simulink model "sm_carousel"  (R2021b)
settings: Solver=ode15s  StartTime=0.0  StopTime=140  MaxStep=0.01  RelTol=1e-3  EnableMultiTasking=on
model workspace (MATLAB code in the model file):
  | oldDir = cd([matlabroot '/toolbox/physmod/sm/smdemos/carousel/initialization']);
  | fparams = @sm_carousel_parameters;
  | cd(oldDir);
  | fparams();
  | clear oldDir fparams;
undefined symbols (not defined in the file): Actrl, sigbuilder_block, Wctrl, X, Y, Z
libraries: sm_carousel_lib x40, sm_lib x30, nesl_utility x7
Description:
  | Fairground Carousel Ride
  | 
  | This example shows a fairground carousel ride. A torque applied to the wheel causes the carousel to rotate and a hydraulic actuator provides the force to lift the arm. The cabs are free to rotate about an axis approximately tangential to the wheel radius. When the wheel is near vertical, the centrifugal acceleration acting on the cabs (caused by the rotation of the wheel) ensures that the cabs are close to a near vertical position. Consequently, the riders are close to 'up-side-down' at the top of the rotation.
  | 
  | The acceleration at the center of the torso of a dummy is measured to show whether the ride is 'fun' and 'safe'. In addition, the hub motor power and hydraulic pressure are measured to validate the design. The control signals (reference and actual) for the hub speed and lift-arm angle are plotted to show the performance of the controllers.
settings Model: Creator=The MathWorks, Inc.  LastModifiedBy=The MathWorks, Inc.
settings SolverCC: AlgebraicLoopSolver=TrustRegion
settings DataIOCC: LimitDataPoints=on  SaveFormat=Array  SaveOutput=off  SignalLogging=off  SaveTime=off  ReturnWorkspaceOutputs=off
settings OptimizationCC: ExpressionDepthLimit=2147483647  LifeSpan=inf
settings DebuggingCC: UnderspecifiedInitializationDetection=Classic  MergeDetectMultiDrivingBlocksExec=none  SolverPrmCheckMsg=warning  StateNameClashWarn=warning  SFUnexpectedBacktrackingDiag=warning  SFNoUnconditionalDefaultTransitionDiag=warning  SFExecutionAtInitializationDiag=none  SFMachineParentedDataDiag=warning  ArithmeticOperatorsInVariantConditions=warning
settings HardwareCC: ProdBitPerPointer=32  ProdBitPerSizeT=32  ProdBitPerPtrDiffT=32  ProdLargestAtomicFloat=None  ProdIntDivRoundTo=Undefined  ProdEndianess=Unspecified  ProdWordSize=32  ProdHWDeviceType=32-bit Generic
settings ModelReferenceCC: PropagateSignalLabelsOutOfModel=off
settings SFSimCC: SimUseLocalCustomCode=off  CustomCodeUndefinedFunction=UseInterfaceOnly
settings RTWCC: RTWUseLocalCustomCode=off
settings CodeAppCC: StateflowObjectComments=on
settings GRTTargetCC: TargetLangStandard=C89/C90 (ANSI)
settings ConfigComp: CovMetricSettings=dw  CovSaveCumulativeToWorkspaceVar=on  CovSaveSingleToWorkspaceVar=on  CovExternalEMLEnable=off  CovSFcnEnable=off
settings SimscapeCC: SimscapeNormalizeSystem=off  SimscapeLogType=all  SimscapeLogSimulationStatistics=on  SimscapeLogName=simlog_sm_carousel  SimscapeLogLimitData=off
settings ConfigurationSet: Description=SimMechanics 2G
settings DiagnosticsConfigSet: SimMechanicsConflictingReferenceFrames=none
settings ExplorerConfigSet: InternalSimMechanicsExplorerSettings="<ExplorerConfiguration><canonicalview>default</canonicalview><TilePanel><TileInfo><Tiles Columns=\"1\" Count=\"1\" Rows=\"1\"><Column Left=\"2\" Weight=\"1\"/><Column Left=\"546\"/><Row Top=\"2\" Weight=\"1\"/><Row Top=\"519\"/><Tile Height=\"1\" Width=\"1\" X=\"0\" Y=\"0\"/></Tiles></TileInfo><SceneInfo><SceneViewer><BGColor><R>0.60000002384185791</R><G>0.60000002384185791</G><B>0.60000002384185791</B></BGColor><Camera><Position><X>22.971265473242269</X><Y>-23.993581807136383</Y><Z>26.226039070736011</Z></Position><Center><X>0.88896183907351589</X><Y>-1.9112781729676298</Y><Z>4.1437354365672574</Z></Center><Up><X>-0.40824829046386307</X><Y>0.40824829046386307</Y><Z>0.81649658092772615</Z></Up><Left>-9.2430366041332803</Left><Right>9.2430366041332803</Right><Bottom>-9.4834843414791639</Bottom><Top>9.4834843414791639</Top></Camera></SceneViewer></SceneInfo></TilePanel></ExplorerConfiguration>"

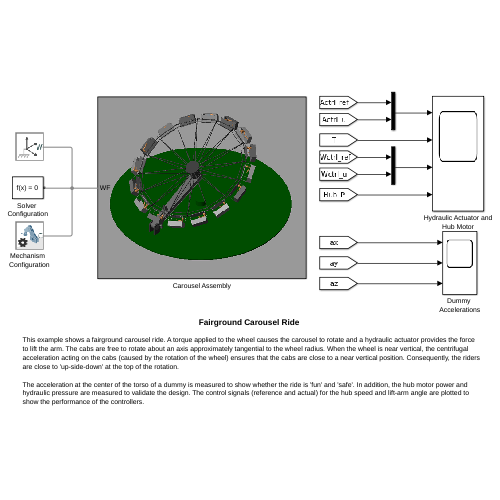
[thumbnail: Simulink's stored preview of the top-level diagram]
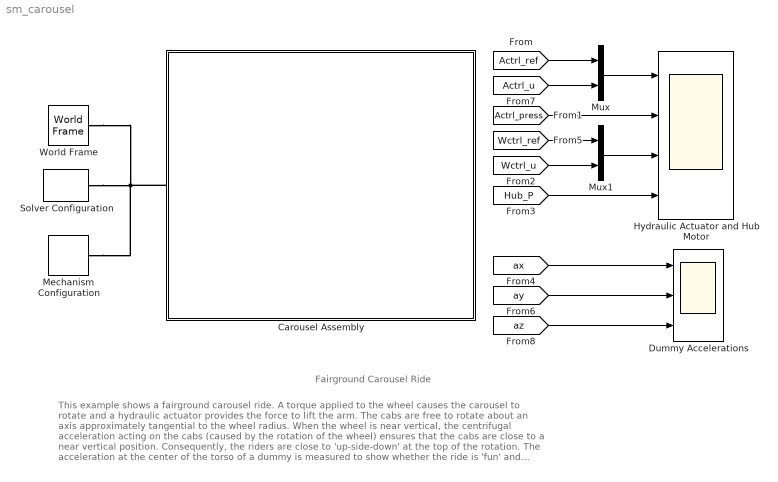
== system sm_carousel ==
  note: This example shows a fairground carousel ride. A torque applied to the wheel causes the carousel to rotate and a hydraulic actuator provides the force
      | to lift the arm. The cabs are free to rotate about an axis approximately tangential to the wheel radius. When the wheel is near vertical, the centrifugal
      | acceleration acting on the cabs (caused by the rotation of the wheel) ensures that the cabs are close to a near vertical position. Consequently, the riders
      | are close to 'up-side-down' at the top of the rotation.
      |
      | The acceleration at the center of the torso of a dummy is measured to show whether the ride is 'fun' and 'safe'. In addition, the hub motor power and
      | hydraulic pressure are measured to validate the design. The control signals (reference and actual) for the hub speed and lift-arm angle are plotted to
      | show the performance of the controllers.
  note: Fairground Carousel Ride
  Carousel Assembly : Subsystem
      mask Display:
      | image(fullfile(matlabroot,'toolbox','physmod','sm','smdemos','carousel','images','sm_carousel.png'));
      | port_label('lconn',1,'WF');
  Dummy Accelerations : Scope  NumInputPorts=3
  Hydraulic Actuator and Hub Motor : Scope  NumInputPorts=4
  Mechanism Configuration : sm_lib/Utilities/Mechanism Configuration  UniformGravity=Constant  GravityVector=[0 0 -9.81]  GravityUnits=m/s^2  LinearizationDelta=0.001  JointModeTransitionNonlinearIterations=2
  Mux : Mux  Inputs=2
  Mux1 : Mux  Inputs=2
  Solver Configuration : nesl_utility/Solver Configuration  PhysicalDomain=network_engine_domain  SubClassName=solver  LeftPortType=input  RightPortType=generic  Tones=[]  Harmonics=[]  SimulateNoise=off  Profile=off  UseLocalSampling=off  EnableSwitchedLinearOptims=on  FrequencyDomain=off  UseCCode=off  RelTol=0.001  AbsTol=1e-06  MinStep=1e-09  ToWorkspace=off  RevertToSquareIcSolve=off  NumHomotopyIterations=100  PhasorMode=off  PhasorModeNumHarmonics=1  DoDC=off  ResidualTolerance=1e-9  UseLocalSolver=off  LocalSolverChoice=NE_BACKWARD_EULER_ADVANCER  LocalSolverSampleTime=.001  DoFixedCost=off  MaxNonlinIter=3  MaxModeIter=2  ComputeImpulses=off  ImpulseIterations=2  LinearAlgebra=Sparse  EquationFormulation=NE_TIME_EF  DelaysMemoryBudget=1024  AutomaticFiltering=on  FilteringTimeConstant=0.001  PartitionStorageMethod=AS_NEEDED  PartitionMemoryBudget=1024  PartitionMethod=FAST
      settings: SourceProductBaseCode=PW,SS
  World Frame : sm_lib/Frames and Transforms/World Frame
  wires:
  [Actrl_ref] -> Mux/1
  [Actrl_u] -> Mux/2
  Mux/1 -> Hydraulic Actuator and Hub Motor/1
  [Wctrl_ref] -> Mux1/1
  [Wctrl_u] -> Mux1/2
  Mux1/1 -> Hydraulic Actuator and Hub Motor/3
  [Actrl_press] -> Hydraulic Actuator and Hub Motor/2
  [Hub_P] -> Hydraulic Actuator and Hub Motor/4
  [az] -> Dummy Accelerations/3
  [ay] -> Dummy Accelerations/2
  [ax] -> Dummy Accelerations/1
  connections:
  Solver Configuration/RConn1 -- Mechanism Configuration/RConn1 -- Carousel Assembly/LConn1 -- World Frame/RConn1

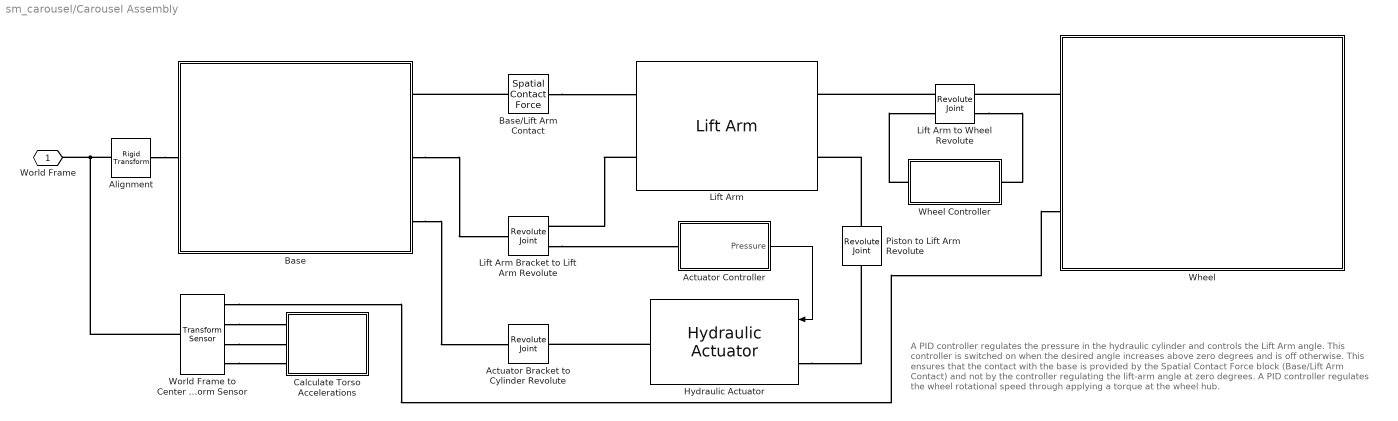
== system sm_carousel/Carousel Assembly ==
  note: A PID controller regulates the pressure in the hydraulic cylinder and controls the Lift Arm angle. This controller is switched on when the desired angle increases above zero degrees and is off otherwise. This ensures that the contact with the base is provided by the Spatial Contact Force block (Base/Lift Arm Contact) and not by the controller regulating the lift-arm angle at zero degrees. A PID controller regulates the wheel rotational speed through applying a torque at the wheel hub.
  Actuator Bracket to Cylinder Revolute : sm_lib/Joints/Revolute Joint  JointMode=Normal  SenseConstraintForce=off  SenseConstraintForceX=off  SenseConstraintForceY=off  SenseConstraintForceZ=off  SenseConstraintTorque=off  SenseConstraintTorqueX=off  SenseConstraintTorqueY=off  SenseConstraintTorqueZ=off  SenseTotalForce=off  SenseTotalForceX=off  SenseTotalForceY=off  SenseTotalForceZ=off  SenseTotalTorque=off  SenseTotalTorqueX=off  SenseTotalTorqueY=off  SenseTotalTorqueZ=off  CompositeWrenchDir=FollowerOnBase  CompositeWrenchFrame=BaseFrame  EquilibriumPosition=0  EquilibriumPositionUnits=deg  SpringStiffness=0  SpringStiffnessUnits=N*m/deg  DampingCoefficient=0  DampingCoefficientUnits=N*m/(deg/s)  TorqueActuationMode=NoTorque  MotionActuationMode=ComputedMotion  SensePosition=off  SenseVelocity=off  SenseAcceleration=off  SenseTorqueForce=off  SenseLowerLimitTorqueForce=off  SenseUpperLimitTorqueForce=off  LowerLimitSpecify=off  LowerLimitBound=-90  LowerLimitBoundUnits=deg  LowerLimitStiffness=1e4  LowerLimitStiffnessUnits=N*m/deg  LowerLimitDamping=10  LowerLimitDampingUnits=N*m/(deg/s)  LowerLimitTransitionRegionWidth=0.1  LowerLimitTransitionRegionWidthUnits=deg  UpperLimitSpecify=off  UpperLimitBound=90  UpperLimitBoundUnits=deg  UpperLimitStiffness=1e4  UpperLimitStiffnessUnits=N*m/deg  UpperLimitDamping=10  UpperLimitDampingUnits=N*m/(deg/s)  UpperLimitTransitionRegionWidth=0.1  UpperLimitTransitionRegionWidthUnits=deg  PositionTargetSpecify=off  PositionTargetPriority=High  PositionTargetValue=0  PositionTargetValueUnits=deg  VelocityTargetSpecify=off  VelocityTargetPriority=High  VelocityTargetValue=0  VelocityTargetValueUnits=deg/s
  Actuator Controller : Subsystem
      mask Display:
      | port_label('lconn',1,'q');
      | port_label('output',1,'P');
  Alignment : sm_lib/Frames and Transforms/Rigid Transform  TranslationMethod=None  TranslationStandardOffset=0  TranslationLengthUnit=m  TranslationStandardAxis=+Z  TranslationCartesianOffset=[0 0 0]  TranslationROffset=0  TranslationROffsetUnits=m  TranslationZOffset=0  TranslationZOffsetUnits=m  TranslationThetaOffset=0  TranslationThetaOffsetUnits=deg  RotationMethod=AlignedAxes  RotationAngleUnits=deg  RotationStandardAxis=+Z  RotationAngle=0  RotationArbitraryAxis=[0 0 1]  FollAlignAxisA=+X  BaseAlignAxisA=+Y  FollAlignAxisB=+Z  BaseAlignAxisB=+Z  RotationSequenceAxes=FollowerAxes  RotationSequence=XYX  RotationSequenceAngles=[0 0 0]  RotationSequenceAnglesUnits=deg  RotationMatrix=[1 0 0; 0 1 0; 0 0 1]
  Base : Subsystem
      mask Display:
      | image(fullfile(matlabroot,'toolbox','physmod','sm','smdemos','carousel','images','sm_carousel_base.png'));
      | port_label('lconn',1,'WF');
      | port_label('rconn',1,'CG');
      | port_label('rconn',2,'RA');
      | port_label('rconn',3,'CB');
  Base/Lift Arm Contact : sm_lib/Forces and Torques/Spatial Contact Force  CoefficientOfDynamicFriction=0.3  CoefficientOfStaticFriction=0.5  SenseContactBaseRotation=off  SenseContactBaseTranslation=off  NormalDamping=Base.b  NormalDampingUnits=N/(m/s)  SenseContactFollowerRotation=off  SenseContactFollowerTranslation=off  SenseContactSignal=off  NormalStiffness=Base.k  NormalStiffnessUnits=N/m  FrictionalCriticalVelocity=1e-3  FrictionalCriticalVelocityUnits=m/s  ZeroCrossDetectContactStartAndEnd=off  FrictionType=None  SenseFrictionalForceMagnitude=off  SenseNormalForceMagnitude=off  NormalForceType=SmoothSpringDamper  SenseNormalVelocity=off  SenseSeparationDistance=off  SenseTangentialVelocity=off  SenseTangentialVelocityMagnitude=off  NormalTransitionRegionWidth=1e-4  NormalTransitionRegionWidthUnits=m
  Calculate Torso Accelerations : Subsystem
      mask Display:
      | port_label('lconn',1,'ax');
      | port_label('lconn',2,'ay');
      | port_label('lconn',3,'az');
  Hydraulic Actuator : sm_carousel_lib/Hydraulic Actuator  Lcyl=Actuator.cyl.Lcyl  Rcyl=Actuator.cyl.Rcyl  Lbase=Actuator.cyl.Lbase  Wbase=Actuator.cyl.Wbase  Rbp=Actuator.cyl.Rbp  Lpist=Actuator.pist.Lpist  Rpist=Actuator.pist.Rpist  Whead=Actuator.pist.Whead  Lhead=Actuator.pist.Lhead  Rhp=Actuator.pist.Rhp  cylColor=Actuator.Mat.cylColor  rhoCyl=Actuator.Mat.rhoCyl  pistColor=Actuator.Mat.pistColor  rhoPist=Actuator.Mat.rhoPist  connColor=Actuator.Mat.connColor  rhoConn=Actuator.Mat.rhoConn
      settings: SourceProductBaseCode=MS
  Lift Arm : sm_carousel_lib/Lift Arm  LiftArmLength=liftArm.ArmMain.ArmLength  rootWidth=liftArm.ArmMain.ArmRootWidth  ArmRadius=liftArm.ArmMain.ArmRadius  LiftArmDepth=liftArm.ArmMain.ArmDepth  LiftArmLip=liftArm.ArmMain.ArmLip  plateThickness=liftArm.ArmMain.Thickness  Hbracket=liftArm.AB.H  Wbracket=liftArm.AB.W  Tbracket=liftArm.AB.T  Dbracket=liftArm.AB.D  Hhole=liftArm.AB.HO  Rhole=liftArm.AB.HR  PistonBracketOffset=liftArm.AB.BO  TopHoleOffset=liftArm.TopPlate.HoleOffset  TopHoleW=liftArm.TopPlate.HoleWidth  TopHoleL=liftArm.TopPlate.HoleLength  BottomHoleOffset=liftArm.BottomPlate.HoleOffset  BottomHoleW=liftArm.BottomPlate.HoleWidth  BottomHoleL=liftArm.BottomPlate.HoleLength  rhoLiftArm=liftArm.ArmMain.Density  LiftArmColor=liftArm.ArmMain.Color
      settings: SourceProductBaseCode=MS
  Lift Arm Bracket to Lift Arm Revolute : sm_lib/Joints/Revolute Joint  JointMode=Normal  SenseConstraintForce=off  SenseConstraintForceX=off  SenseConstraintForceY=off  SenseConstraintForceZ=off  SenseConstraintTorque=off  SenseConstraintTorqueX=off  SenseConstraintTorqueY=off  SenseConstraintTorqueZ=off  SenseTotalForce=off  SenseTotalForceX=off  SenseTotalForceY=off  SenseTotalForceZ=off  SenseTotalTorque=off  SenseTotalTorqueX=off  SenseTotalTorqueY=off  SenseTotalTorqueZ=off  CompositeWrenchDir=FollowerOnBase  CompositeWrenchFrame=BaseFrame  EquilibriumPosition=0  EquilibriumPositionUnits=deg  SpringStiffness=0  SpringStiffnessUnits=N*m/deg  DampingCoefficient=0  DampingCoefficientUnits=N*m/(deg/s)  TorqueActuationMode=NoTorque  MotionActuationMode=ComputedMotion  SensePosition=on  SenseVelocity=off  SenseAcceleration=off  SenseTorqueForce=off  SenseLowerLimitTorqueForce=off  SenseUpperLimitTorqueForce=off  LowerLimitSpecify=off  LowerLimitBound=-90  LowerLimitBoundUnits=deg  LowerLimitStiffness=1e4  LowerLimitStiffnessUnits=N*m/deg  LowerLimitDamping=10  LowerLimitDampingUnits=N*m/(deg/s)  LowerLimitTransitionRegionWidth=0.1  LowerLimitTransitionRegionWidthUnits=deg  UpperLimitSpecify=off  UpperLimitBound=90  UpperLimitBoundUnits=deg  UpperLimitStiffness=1e4  UpperLimitStiffnessUnits=N*m/deg  UpperLimitDamping=10  UpperLimitDampingUnits=N*m/(deg/s)  UpperLimitTransitionRegionWidth=0.1  UpperLimitTransitionRegionWidthUnits=deg  PositionTargetSpecify=on  PositionTargetPriority=High  PositionTargetValue=liftArm.Revolute.InitAngle  PositionTargetValueUnits=deg  VelocityTargetSpecify=off  VelocityTargetPriority=High  VelocityTargetValue=0  VelocityTargetValueUnits=deg/s
  Lift Arm to Wheel Revolute : sm_lib/Joints/Revolute Joint  JointMode=Normal  SenseConstraintForce=off  SenseConstraintForceX=off  SenseConstraintForceY=off  SenseConstraintForceZ=off  SenseConstraintTorque=off  SenseConstraintTorqueX=off  SenseConstraintTorqueY=off  SenseConstraintTorqueZ=off  SenseTotalForce=off  SenseTotalForceX=off  SenseTotalForceY=off  SenseTotalForceZ=off  SenseTotalTorque=off  SenseTotalTorqueX=off  SenseTotalTorqueY=off  SenseTotalTorqueZ=off  CompositeWrenchDir=FollowerOnBase  CompositeWrenchFrame=BaseFrame  EquilibriumPosition=0  EquilibriumPositionUnits=deg  SpringStiffness=0  SpringStiffnessUnits=N*m/deg  DampingCoefficient=0  DampingCoefficientUnits=N*m/(deg/s)  TorqueActuationMode=InputTorque  MotionActuationMode=ComputedMotion  SensePosition=off  SenseVelocity=on  SenseAcceleration=off  SenseTorqueForce=off  SenseLowerLimitTorqueForce=off  SenseUpperLimitTorqueForce=off  LowerLimitSpecify=off  LowerLimitBound=-90  LowerLimitBoundUnits=deg  LowerLimitStiffness=1e4  LowerLimitStiffnessUnits=N*m/deg  LowerLimitDamping=10  LowerLimitDampingUnits=N*m/(deg/s)  LowerLimitTransitionRegionWidth=0.1  LowerLimitTransitionRegionWidthUnits=deg  UpperLimitSpecify=off  UpperLimitBound=90  UpperLimitBoundUnits=deg  UpperLimitStiffness=1e4  UpperLimitStiffnessUnits=N*m/deg  UpperLimitDamping=10  UpperLimitDampingUnits=N*m/(deg/s)  UpperLimitTransitionRegionWidth=0.1  UpperLimitTransitionRegionWidthUnits=deg  PositionTargetSpecify=off  PositionTargetPriority=High  PositionTargetValue=0  PositionTargetValueUnits=deg  VelocityTargetSpecify=off  VelocityTargetPriority=High  VelocityTargetValue=0  VelocityTargetValueUnits=deg/s
  Piston to Lift Arm Revolute : sm_lib/Joints/Revolute Joint  JointMode=Normal  SenseConstraintForce=off  SenseConstraintForceX=off  SenseConstraintForceY=off  SenseConstraintForceZ=off  SenseConstraintTorque=off  SenseConstraintTorqueX=off  SenseConstraintTorqueY=off  SenseConstraintTorqueZ=off  SenseTotalForce=off  SenseTotalForceX=off  SenseTotalForceY=off  SenseTotalForceZ=off  SenseTotalTorque=off  SenseTotalTorqueX=off  SenseTotalTorqueY=off  SenseTotalTorqueZ=off  CompositeWrenchDir=FollowerOnBase  CompositeWrenchFrame=BaseFrame  EquilibriumPosition=0  EquilibriumPositionUnits=deg  SpringStiffness=0  SpringStiffnessUnits=N*m/deg  DampingCoefficient=0  DampingCoefficientUnits=N*m/(deg/s)  TorqueActuationMode=NoTorque  MotionActuationMode=ComputedMotion  SensePosition=off  SenseVelocity=off  SenseAcceleration=off  SenseTorqueForce=off  SenseLowerLimitTorqueForce=off  SenseUpperLimitTorqueForce=off  LowerLimitSpecify=off  LowerLimitBound=-90  LowerLimitBoundUnits=deg  LowerLimitStiffness=1e4  LowerLimitStiffnessUnits=N*m/deg  LowerLimitDamping=10  LowerLimitDampingUnits=N*m/(deg/s)  LowerLimitTransitionRegionWidth=0.1  LowerLimitTransitionRegionWidthUnits=deg  UpperLimitSpecify=off  UpperLimitBound=90  UpperLimitBoundUnits=deg  UpperLimitStiffness=1e4  UpperLimitStiffnessUnits=N*m/deg  UpperLimitDamping=10  UpperLimitDampingUnits=N*m/(deg/s)  UpperLimitTransitionRegionWidth=0.1  UpperLimitTransitionRegionWidthUnits=deg  PositionTargetSpecify=off  PositionTargetPriority=High  PositionTargetValue=0  PositionTargetValueUnits=deg  VelocityTargetSpecify=off  VelocityTargetPriority=High  VelocityTargetValue=0  VelocityTargetValueUnits=deg/s
  Wheel : Subsystem
      mask Display:
      | image(fullfile(matlabroot,'toolbox','physmod','sm','smdemos','carousel','images','sm_carousel_wheel_assembly.png'));
      | port_label('lconn',2,'CT');
      | port_label('lconn',1,'HA');
  Wheel Controller : Subsystem
      mask Display:
      | port_label('rconn',1,'T');
      | port_label('lconn',1,'w');
  World Frame to Center Torso XForm Sensor : sm_lib/Frames and Transforms/Transform Sensor  MeasurementFrame=NonRotatingFollower  SenseAngle=off  SenseAxis=off  SenseAngle1=off  SenseAngle2=off  SenseAngle3=off  SenseQ=off  SenseR=off  SenseOmegaX=off  SenseOmegaY=off  SenseOmegaZ=off  SenseOmega1=off  SenseOmega2=off  SenseOmega3=off  SenseQDot=off  SenseRDot=off  SenseAlphaX=off  SenseAlphaY=off  SenseAlphaZ=off  SenseAlpha1=off  SenseAlpha2=off  SenseAlpha3=off  SenseQDDot=off  SenseRDDot=off  SenseX=off  SenseY=off  SenseZ=off  SenseRad=off  SenseAzim=off  SenseDist=off  SenseInc=off  SenseXDot=off  SenseYDot=off  SenseZDot=off  SenseRadDot=off  SenseAzimDot=off  SenseDistDot=off  SenseIncDot=off  SenseXDDot=on  SenseYDDot=on  SenseZDDot=on  SenseRadDDot=off  SenseAzimDDot=off  SenseDistDDot=off  SenseIncDDot=off
  World Frame : PMIOPort  Side=Left
  wires:
  Actuator Controller/1(Pressure) -> Hydraulic Actuator/1
  connections:
  Base/RConn3 -- Actuator Bracket to Cylinder Revolute/LConn1
  Lift Arm Bracket to Lift Arm Revolute/RConn2 -- Actuator Controller/LConn1
  Wheel Controller/RConn1 -- Lift Arm to Wheel Revolute/LConn2
  Base/RConn2 -- Lift Arm Bracket to Lift Arm Revolute/LConn1
  Lift Arm/LConn2 -- Lift Arm Bracket to Lift Arm Revolute/RConn1
  Hydraulic Actuator/LConn1 -- Piston to Lift Arm Revolute/LConn1
  Lift Arm to Wheel Revolute/LConn1 -- Lift Arm/RConn1
  Piston to Lift Arm Revolute/RConn1 -- Lift Arm/RConn2
  Hydraulic Actuator/RConn1 -- Actuator Bracket to Cylinder Revolute/RConn1
  World Frame to Center Torso XForm Sensor/RConn1 -- Wheel/LConn2
  World Frame to Center Torso XForm Sensor/LConn1 -- Alignment/LConn1 -- World Frame/RConn1
  Lift Arm to Wheel Revolute/RConn2 -- Wheel Controller/LConn1
  World Frame to Center Torso XForm Sensor/RConn2 -- Calculate Torso Accelerations/LConn1
  World Frame to Center Torso XForm Sensor/RConn3 -- Calculate Torso Accelerations/LConn2
  World Frame to Center Torso XForm Sensor/RConn4 -- Calculate Torso Accelerations/LConn3
  Wheel/LConn1 -- Lift Arm to Wheel Revolute/RConn1
  Alignment/RConn1 -- Base/LConn1
  Base/Lift Arm Contact/LConn1 -- Base/RConn1
  Base/Lift Arm Contact/RConn1 -- Lift Arm/LConn1

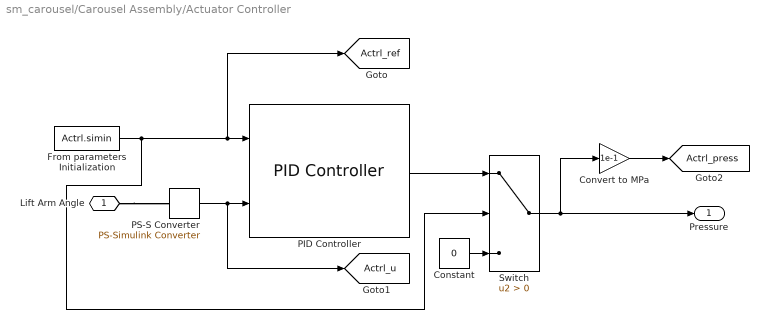
== system sm_carousel/Carousel Assembly/Actuator Controller ==
  Constant : Constant  Value=0
  Convert to MPa : Gain  Gain=1e-1
  From parameters Initialization : FromWorkspace  VariableName=Actrl.simin
  PID Controller : sm_carousel_lib/PID Controller  Kp=Actrl.kp  Ki=Actrl.ki  Kd=Actrl.kd  N=Actrl.N
      settings: SourceProductBaseCode=MS
  PS-S Converter : nesl_utility/PS-Simulink Converter  PhysicalDomain=network_engine_domain  SubClassName=ps_output  LeftPortType=input  RightPortType=output  PseudoPeriodic=off  Frequencies=[]  Unit=deg  AffineConversion=off
      settings: SourceProductBaseCode=PW,SS
  Switch : Switch  Criteria=u2 > Threshold
  Lift Arm Angle : PMIOPort  Side=Left
  Pressure : Outport
  tag scope: Actrl_press=global, Actrl_ref=global, Actrl_u=global
  wires:
  PS-S Converter/1 -> PID Controller/2, [Actrl_u]
  Convert to MPa/1 -> [Actrl_press]
  Switch/1 -> Pressure/1, Convert to MPa/1
  PID Controller/1 -> Switch/1
  Constant/1 -> Switch/3
  From parameters Initialization/1 -> Switch/2, [Actrl_ref], PID Controller/1
  connections:
  Lift Arm Angle/RConn1 -- PS-S Converter/LConn1

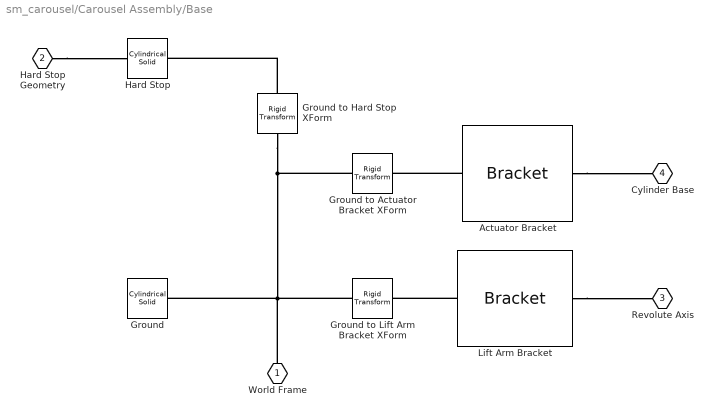
== system sm_carousel/Carousel Assembly/Base ==
  Actuator Bracket : sm_carousel_lib/Bracket  Hbracket=Base.AB.H  Wbracket=Base.AB.W  Tbracket=Base.AB.T  Dbracket=Base.AB.D  Hhole=Base.AB.HH  Rhole=Base.AB.RH  rhoBracket=Base.AB.RHO  bracketColor=Base.AB.COLOR
      settings: SourceProductBaseCode=MS
  Ground : sm_lib/Body Elements/Cylindrical Solid  GraphicAmbientColor=[0.15 0.15 0.15 1.0]  BasedOnType=Density  CenterOfMass=[0 0 0]  CenterOfMassUnits=m  GraphicDiffuseColor=Base.Color  CylinderLength=Base.Ground.t  CylinderLengthUnits=m  CylinderRadius=Base.Ground.r  CylinderRadiusUnits=m  Density=1000  DensityUnits=kg/(m^3)  DoExposeReferenceFrame=on  GraphicEmissiveColor=[0.0 0.0 0.0 1.0]  ExportEntireGeometry=off  SerializedFrames=<Frames/>  MarkerShape=Sphere  MarkerSize=10  GraphicType=FromGeometry  InertiaType=CalculateFromGeometry  Mass=1  MassUnits=kg  MomentsOfInertia=[1 1 1]  MomentsOfInertiaUnits=kg*m^2  GraphicOpacity=1.0  ProductsOfInertia=[0 0 0]  ProductsOfInertiaUnits=kg*m^2  GraphicShininess=75  GraphicSpecularColor=[0.5 0.5 0.5 1.0]  GraphicVisPropType=SimpleVisualProperties
  Ground to Hard Stop XForm : sm_lib/Frames and Transforms/Rigid Transform  TranslationMethod=Cartesian  TranslationStandardOffset=0  TranslationLengthUnit=m  TranslationStandardAxis=+Z  TranslationCartesianOffset=Base.HardStop.Offset  TranslationROffset=0  TranslationROffsetUnits=m  TranslationZOffset=0  TranslationZOffsetUnits=m  TranslationThetaOffset=0  TranslationThetaOffsetUnits=deg  RotationMethod=None  RotationAngleUnits=deg  RotationStandardAxis=+Z  RotationAngle=0  RotationArbitraryAxis=[0 0 1]  FollAlignAxisA=+X  BaseAlignAxisA=+Y  FollAlignAxisB=+Y  BaseAlignAxisB=+Z  RotationSequenceAxes=FollowerAxes  RotationSequence=XYX  RotationSequenceAngles=[0 0 0]  RotationSequenceAnglesUnits=deg  RotationMatrix=[1 0 0; 0 1 0; 0 0 1]
  Ground to Actuator Bracket XForm : sm_lib/Frames and Transforms/Rigid Transform  TranslationMethod=Cartesian  TranslationStandardOffset=0  TranslationLengthUnit=m  TranslationStandardAxis=+Z  TranslationCartesianOffset=Base.AB.Offset  TranslationROffset=0  TranslationROffsetUnits=m  TranslationZOffset=0  TranslationZOffsetUnits=m  TranslationThetaOffset=0  TranslationThetaOffsetUnits=deg  RotationMethod=AlignedAxes  RotationAngleUnits=deg  RotationStandardAxis=+Z  RotationAngle=0  RotationArbitraryAxis=[0 0 1]  FollAlignAxisA=-Y  BaseAlignAxisA=+Y  FollAlignAxisB=-X  BaseAlignAxisB=+X  RotationSequenceAxes=FollowerAxes  RotationSequence=XYX  RotationSequenceAngles=[0 0 0]  RotationSequenceAnglesUnits=deg  RotationMatrix=[1 0 0; 0 1 0; 0 0 1]
  Ground to Lift Arm Bracket XForm : sm_lib/Frames and Transforms/Rigid Transform  TranslationMethod=Cartesian  TranslationStandardOffset=0  TranslationLengthUnit=m  TranslationStandardAxis=+X  TranslationCartesianOffset=Base.LAB.Offset  TranslationROffset=0  TranslationROffsetUnits=m  TranslationZOffset=0  TranslationZOffsetUnits=m  TranslationThetaOffset=0  TranslationThetaOffsetUnits=deg  RotationMethod=None  RotationAngleUnits=deg  RotationStandardAxis=+Z  RotationAngle=0  RotationArbitraryAxis=[0 0 1]  FollAlignAxisA=+X  BaseAlignAxisA=-Y  FollAlignAxisB=+Y  BaseAlignAxisB=+X  RotationSequenceAxes=FollowerAxes  RotationSequence=XYX  RotationSequenceAngles=[0 0 0]  RotationSequenceAnglesUnits=deg  RotationMatrix=[1 0 0; 0 1 0; 0 0 1]
  Hard Stop : sm_lib/Body Elements/Cylindrical Solid  GraphicAmbientColor=[0.15 0.15 0.15 1.0]  BasedOnType=Density  CenterOfMass=[0 0 0]  CenterOfMassUnits=m  GraphicDiffuseColor=Base.Color  CylinderLength=Base.HardStop.Depth  CylinderLengthUnits=m  CylinderRadius=Base.HardStop.r  CylinderRadiusUnits=m  Density=1000  DensityUnits=kg/(m^3)  DoExposeReferenceFrame=on  GraphicEmissiveColor=[0.0 0.0 0.0 1.0]  ExportEntireGeometry=on  SerializedFrames=<Frames/>  MarkerShape=Sphere  MarkerSize=10  GraphicType=FromGeometry  InertiaType=CalculateFromGeometry  Mass=1  MassUnits=kg  MomentsOfInertia=[1 1 1]  MomentsOfInertiaUnits=kg*m^2  GraphicOpacity=1.0  ProductsOfInertia=[0 0 0]  ProductsOfInertiaUnits=kg*m^2  GraphicShininess=75  GraphicSpecularColor=[0.5 0.5 0.5 1.0]  GraphicVisPropType=SimpleVisualProperties
  Lift Arm Bracket : sm_carousel_lib/Bracket  Hbracket=Base.LAB.H  Wbracket=Base.LAB.W  Tbracket=Base.LAB.T  Dbracket=Base.LAB.D  Hhole=Base.LAB.HH  Rhole=Base.LAB.RH  rhoBracket=Base.LAB.RHO  bracketColor=Base.LAB.COLOR
      settings: SourceProductBaseCode=MS
  World Frame : PMIOPort  Side=Left
  Hard Stop Geometry : PMIOPort  Port=2  Side=Right
  Revolute Axis : PMIOPort  Port=3  Side=Right
  Cylinder Base : PMIOPort  Port=4  Side=Right
  connections:
  Ground to Hard Stop XForm/RConn1 -- Hard Stop/RConn1
  Ground to Hard Stop XForm/LConn1 -- Ground to Actuator Bracket XForm/LConn1 -- Ground to Lift Arm Bracket XForm/LConn1 -- World Frame/RConn1 -- Ground/RConn1
  Lift Arm Bracket/LConn1 -- Ground to Lift Arm Bracket XForm/RConn1
  Lift Arm Bracket/RConn1 -- Revolute Axis/RConn1
  Actuator Bracket/LConn1 -- Ground to Actuator Bracket XForm/RConn1
  Actuator Bracket/RConn1 -- Cylinder Base/RConn1
  Hard Stop Geometry/RConn1 -- Hard Stop/LConn1

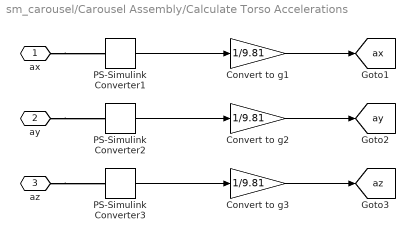
== system sm_carousel/Carousel Assembly/Calculate Torso Accelerations ==
  Convert to g1 : Gain  Gain=1/9.81
  Convert to g2 : Gain  Gain=1/9.81
  Convert to g3 : Gain  Gain=1/9.81
  PS-Simulink Converter1 : nesl_utility/PS-Simulink Converter  PhysicalDomain=network_engine_domain  SubClassName=ps_output  LeftPortType=input  RightPortType=output  PseudoPeriodic=off  Frequencies=[]  Unit=1  AffineConversion=off
      settings: SourceProductBaseCode=PW,SS
  PS-Simulink Converter2 : nesl_utility/PS-Simulink Converter  PhysicalDomain=network_engine_domain  SubClassName=ps_output  LeftPortType=input  RightPortType=output  PseudoPeriodic=off  Frequencies=[]  Unit=1  AffineConversion=off
      settings: SourceProductBaseCode=PW,SS
  PS-Simulink Converter3 : nesl_utility/PS-Simulink Converter  PhysicalDomain=network_engine_domain  SubClassName=ps_output  LeftPortType=input  RightPortType=output  PseudoPeriodic=off  Frequencies=[]  Unit=1  AffineConversion=off
      settings: SourceProductBaseCode=PW,SS
  ax : PMIOPort  Side=Left
  ay : PMIOPort  Port=2  Side=Left
  az : PMIOPort  Port=3  Side=Left
  tag scope: ax=global, ay=global, az=global
  wires:
  PS-Simulink Converter3/1 -> Convert to g3/1
  PS-Simulink Converter2/1 -> Convert to g2/1
  PS-Simulink Converter1/1 -> Convert to g1/1
  Convert to g1/1 -> [ax]
  Convert to g2/1 -> [ay]
  Convert to g3/1 -> [az]
  connections:
  ay/RConn1 -- PS-Simulink Converter2/LConn1
  ax/RConn1 -- PS-Simulink Converter1/LConn1
  az/RConn1 -- PS-Simulink Converter3/LConn1

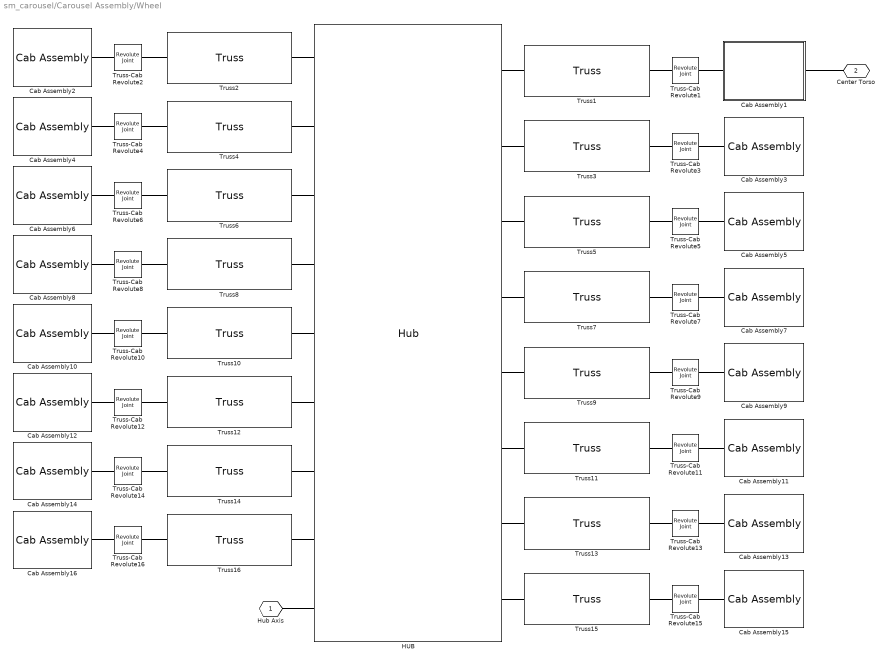
== system sm_carousel/Carousel Assembly/Wheel ==
  Cab Assembly1 : Subsystem
      mask Display:
      | image(fullfile(matlabroot,'toolbox','physmod','sm','smdemos','carousel','images','sm_carousel_cab_assembly.png'));
      | port_label('lconn',1,'CC');
      | port_label('rconn',1,'CT');
  Cab Assembly{2,4,6,8,10,12,14,16} (8 alike) : sm_carousel_lib/Cab Assembly  CabLength=Cab.Length  CabWidth=Cab.Width  CabPlateThickness=Cab.PlateThickness  CabBodyConnW=Cab.BodyConnW  CabBodyConnH=Cab.BodyConnH  CabWindowHeight=Cab.WindowHeight  SpacerThickness=Cab.WindowColumnThickness  CabTubDepth=Cab.TubDepth  RP_CD=Cab.RP.CD  RP_W=Cab.RP.W  RP_H=Cab.RP.H  RP_TL=Cab.RP.TL  RP_HR=Cab.RP.HR  RP_PT=Cab.RP.PT  RP_HO=Cab.RP.HO  DummyHeight=Cab.Dummy.Height  DummyDensity=Cab.Dummy.Density  rhoCab=Cab.Density  CabColor=Cab.ColorB
      settings: SourceProductBaseCode=MS
  Cab Assembly{3,5,7,9,11,13,15} (7 alike) : sm_carousel_lib/Cab Assembly  CabLength=Cab.Length  CabWidth=Cab.Width  CabPlateThickness=Cab.PlateThickness  CabBodyConnW=Cab.BodyConnW  CabBodyConnH=Cab.BodyConnH  CabWindowHeight=Cab.WindowHeight  SpacerThickness=Cab.WindowColumnThickness  CabTubDepth=Cab.TubDepth  RP_CD=Cab.RP.CD  RP_W=Cab.RP.W  RP_H=Cab.RP.H  RP_TL=Cab.RP.TL  RP_HR=Cab.RP.HR  RP_PT=Cab.RP.PT  RP_HO=Cab.RP.HO  DummyHeight=Cab.Dummy.Height  DummyDensity=Cab.Dummy.Density  rhoCab=Cab.Density  CabColor=Cab.ColorA
      settings: SourceProductBaseCode=MS
  HUB : sm_carousel_lib/Hub  HubOuterRadius=Hub.OuterRadius  HubThickness=Hub.Thickness  HubDepth=Hub.Depth  HubCapRadius=Hub.CapRadius  HubCapThickness=Hub.CapThickness  nCabs=Hub.nCabs  rho=Hub.Density  HubColor=Hub.Color
      settings: SourceProductBaseCode=MS
  Truss-Cab Revolute{1..16} (16 alike) : sm_lib/Joints/Revolute Joint  JointMode=Normal  SenseConstraintForce=off  SenseConstraintForceX=off  SenseConstraintForceY=off  SenseConstraintForceZ=off  SenseConstraintTorque=off  SenseConstraintTorqueX=off  SenseConstraintTorqueY=off  SenseConstraintTorqueZ=off  SenseTotalForce=off  SenseTotalForceX=off  SenseTotalForceY=off  SenseTotalForceZ=off  SenseTotalTorque=off  SenseTotalTorqueX=off  SenseTotalTorqueY=off  SenseTotalTorqueZ=off  CompositeWrenchDir=FollowerOnBase  CompositeWrenchFrame=BaseFrame  EquilibriumPosition=0  EquilibriumPositionUnits=deg  SpringStiffness=0  SpringStiffnessUnits=N*m/deg  DampingCoefficient=Cab.joint.damping  DampingCoefficientUnits=N*m/(deg/s)  TorqueActuationMode=NoTorque  MotionActuationMode=ComputedMotion  SensePosition=off  SenseVelocity=off  SenseAcceleration=off  SenseTorqueForce=off  SenseLowerLimitTorqueForce=off  SenseUpperLimitTorqueForce=off  LowerLimitSpecify=off  LowerLimitBound=-90  LowerLimitBoundUnits=deg  LowerLimitStiffness=1e4  LowerLimitStiffnessUnits=N*m/deg  LowerLimitDamping=10  LowerLimitDampingUnits=N*m/(deg/s)  LowerLimitTransitionRegionWidth=0.1  LowerLimitTransitionRegionWidthUnits=deg  UpperLimitSpecify=off  UpperLimitBound=90  UpperLimitBoundUnits=deg  UpperLimitStiffness=1e4  UpperLimitStiffnessUnits=N*m/deg  UpperLimitDamping=10  UpperLimitDampingUnits=N*m/(deg/s)  UpperLimitTransitionRegionWidth=0.1  UpperLimitTransitionRegionWidthUnits=deg  PositionTargetSpecify=off  PositionTargetPriority=High  PositionTargetValue=0  PositionTargetValueUnits=deg  VelocityTargetSpecify=off  VelocityTargetPriority=High  VelocityTargetValue=0  VelocityTargetValueUnits=deg/s
  Truss{1..16} (16 alike) : sm_carousel_lib/Truss  RootDepth=Truss.RootDepth  TrussLength=Truss.ArmLength  MemberWidth=Truss.memberWidth  MemberThickness=Truss.memberThickness  BraceLength=Truss.braceLength  BraceAngle=Truss.braceAngle  EPConnectionDepth=Truss.EP.CD  EPWidth=Truss.EP.W  EPHeight=Truss.EP.H  EPTaperedLength=Truss.EP.TL  EPHoleRadius=Truss.EP.HR  EPThickness=Truss.EP.T  EPHoleOffset=Truss.EP.HO  PinAngle=Truss.pin.Angle  PinOuterRadius=Truss.pin.OuterRadius  PinThickness=Truss.pin.Thickness  PinLength=Truss.pin.Length  rhoTruss=Truss.Density  TrussColor=Truss.Color
      settings: SourceProductBaseCode=MS
  Hub Axis : PMIOPort  Side=Left
  Center Torso : PMIOPort  Port=2  Side=Left
  connections:
  HUB/RConn1 -- Truss1/LConn1
  Truss1/RConn1 -- Truss-Cab Revolute1/LConn1
  Truss2/RConn1 -- Truss-Cab Revolute2/LConn1
  Truss-Cab Revolute2/RConn1 -- Cab Assembly2/LConn1
  Truss-Cab Revolute4/RConn1 -- Cab Assembly4/LConn1
  Truss4/RConn1 -- Truss-Cab Revolute4/LConn1
  Truss6/RConn1 -- Truss-Cab Revolute6/LConn1
  Truss-Cab Revolute6/RConn1 -- Cab Assembly6/LConn1
  Truss-Cab Revolute3/RConn1 -- Cab Assembly3/LConn1
  Truss3/RConn1 -- Truss-Cab Revolute3/LConn1
  Truss5/RConn1 -- Truss-Cab Revolute5/LConn1
  Truss-Cab Revolute5/RConn1 -- Cab Assembly5/LConn1
  Truss-Cab Revolute7/RConn1 -- Cab Assembly7/LConn1
  Truss7/RConn1 -- Truss-Cab Revolute7/LConn1
  Truss-Cab Revolute8/RConn1 -- Cab Assembly8/LConn1
  Truss8/RConn1 -- Truss-Cab Revolute8/LConn1
  Truss-Cab Revolute9/RConn1 -- Cab Assembly9/LConn1
  Truss9/RConn1 -- Truss-Cab Revolute9/LConn1
  Truss10/RConn1 -- Truss-Cab Revolute10/LConn1
  Truss-Cab Revolute10/RConn1 -- Cab Assembly10/LConn1
  Truss11/RConn1 -- Truss-Cab Revolute11/LConn1
  Truss-Cab Revolute11/RConn1 -- Cab Assembly11/LConn1
  Truss-Cab Revolute12/RConn1 -- Cab Assembly12/LConn1
  Truss12/RConn1 -- Truss-Cab Revolute12/LConn1
  Truss-Cab Revolute13/RConn1 -- Cab Assembly13/LConn1
  Truss13/RConn1 -- Truss-Cab Revolute13/LConn1
  Truss14/RConn1 -- Truss-Cab Revolute14/LConn1
  Truss-Cab Revolute14/RConn1 -- Cab Assembly14/LConn1
  Truss15/RConn1 -- Truss-Cab Revolute15/LConn1
  Truss-Cab Revolute15/RConn1 -- Cab Assembly15/LConn1
  Truss-Cab Revolute16/RConn1 -- Cab Assembly16/LConn1
  Truss16/RConn1 -- Truss-Cab Revolute16/LConn1
  HUB/RConn2 -- Truss3/LConn1
  HUB/RConn3 -- Truss5/LConn1
  HUB/RConn4 -- Truss7/LConn1
  HUB/RConn5 -- Truss9/LConn1
  HUB/RConn6 -- Truss11/LConn1
  HUB/RConn7 -- Truss13/LConn1
  HUB/RConn8 -- Truss15/LConn1
  Truss2/LConn1 -- HUB/LConn1
  Truss4/LConn1 -- HUB/LConn2
  Truss6/LConn1 -- HUB/LConn3
  Truss8/LConn1 -- HUB/LConn4
  Truss10/LConn1 -- HUB/LConn5
  Truss12/LConn1 -- HUB/LConn6
  Truss14/LConn1 -- HUB/LConn7
  Truss16/LConn1 -- HUB/LConn8
  HUB/LConn9 -- Hub Axis/RConn1
  Cab Assembly1/LConn1 -- Truss-Cab Revolute1/RConn1
  Center Torso/RConn1 -- Cab Assembly1/RConn1

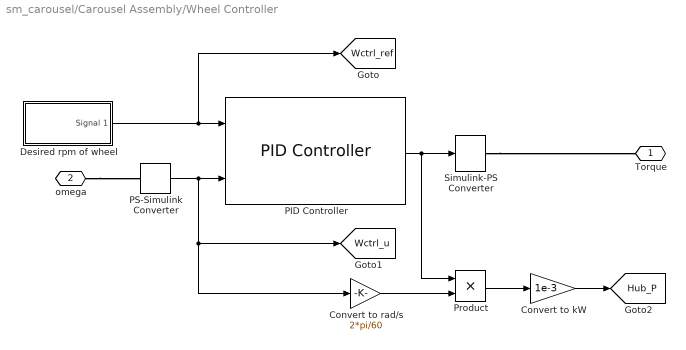
== system sm_carousel/Carousel Assembly/Wheel Controller ==
  Convert to kW : Gain  Gain=1e-3
  Convert to rad/s : Gain  Gain=2*pi/60
  Desired rpm of wheel : Subsystem  Tag=STV Subsys  LoadFcn=sigbuilder_block('load');  StartFcn=sigbuilder_block('start');  StopFcn=sigbuilder_block('stop');  ClipboardFcn=sigbuilder_block('clipboard');  mask(Sigbuilder block){tuvar=[0:10]}
      mask help: Simulink:masks:SigbuilderBlock_MD
      mask init:
      | if ~strcmp(get_param(bdroot(gcbh),'SimulationStatus'),'stopped') tuvar = sigbuilder_block('maskInit'); end
      settings: CopyFcn=sigbuilder_block('copy');  DeleteFcn=sigbuilder_block('delete');  ModelCloseFcn=sigbuilder_block('modelClose');  PreSaveFcn=sigbuilder_block('preSave');  PauseFcn=sigbuilder_block('pause');  ContinueFcn=sigbuilder_block('continue');  NameChangeFcn=sigbuilder_block('namechange');  OpenFcn=sigbuilder_block('open',[709.5 69 683.25 489.75 ]);  CloseFcn=sigbuilder_block('close');
      mask Display: plot(0, 0, 100, 100,[2, 2, 32, 32, 2], [68, 8, 8, 68, 68],[32, 2], [38, 38], [32, 19, 2],[53, 60, 44], [32, 17, 17, 2],[16, 16, 31, 31]);txt = getActiveGroup(gcbh);text(2, 100, txt,'verticalAlignment', 'top');
  PID Controller : sm_carousel_lib/PID Controller  Kp=Wctrl.kp  Ki=Wctrl.ki  Kd=Wctrl.kd  N=Wctrl.N
      settings: SourceProductBaseCode=MS
  PS-Simulink Converter : nesl_utility/PS-Simulink Converter  PhysicalDomain=network_engine_domain  SubClassName=ps_output  LeftPortType=input  RightPortType=output  PseudoPeriodic=off  Frequencies=[]  Unit=rpm  AffineConversion=off
      settings: SourceProductBaseCode=PW,SS
  Product : Product  RndMeth=Zero
  Simulink-PS Converter : nesl_utility/Simulink-PS Converter  PhysicalDomain=network_engine_domain  SubClassName=ps_input  LeftPortType=input  RightPortType=output  PseudoPeriodic=off  Frequencies=[]  NoiseDistribution=none  NoiseParameters=[]  Unit=1  AffineConversion=off  FilteringAndDerivatives=zero  SimscapeFilterOrder=1  InputFilterTimeConstant=.001  UdotUserProvided=1
      settings: SourceProductBaseCode=PW,SS
  Torque : PMIOPort  Side=Right
  omega : PMIOPort  Port=2  Side=Left
  tag scope: Hub_P=global, Wctrl_ref=global, Wctrl_u=global
  wires:
  Desired rpm of wheel/1(Signal 1) -> [Wctrl_ref], PID Controller/1
  PS-Simulink Converter/1 -> [Wctrl_u], Convert to rad/s/1, PID Controller/2
  PID Controller/1 -> Product/1, Simulink-PS Converter/1
  Product/1 -> Convert to kW/1
  Convert to rad/s/1 -> Product/2
  Convert to kW/1 -> [Hub_P]
  connections:
  omega/RConn1 -- PS-Simulink Converter/LConn1
  Simulink-PS Converter/RConn1 -- Torque/RConn1

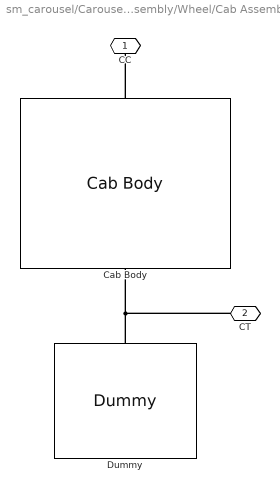
== system sm_carousel/Carousel Assembly/Wheel/Cab Assembly1 ==
  Cab Body : sm_carousel_lib/Cab Body  CabLength=Cab.Length  CabWidth=Cab.Width  PlateThickness=Cab.PlateThickness  ConnectorWidth=Cab.BodyConnW  ConnectorHeight=Cab.BodyConnH  SpacerHeight=Cab.WindowHeight  SpacerThickness=Cab.WindowColumnThickness  TubDepth=Cab.TubDepth  RP_CD=Cab.RP.CD  RP_W=Cab.RP.W  RP_H=Cab.RP.H  RP_TL=Cab.RP.TL  RP_HR=Cab.RP.HR  RP_PT=Cab.RP.PT  RP_HO=Cab.RP.HO  rhoCab=Cab.Density  CabColor=Cab.ColorA
      settings: SourceProductBaseCode=MS
  Dummy : sm_carousel_lib/Dummy  height=Cab.Dummy.Height  personDensity=Cab.Dummy.Density
      settings: SourceProductBaseCode=MS
  CC : PMIOPort  Side=Left
  CT : PMIOPort  Port=2  Side=Right
  connections:
  Cab Body/LConn1 -- CC/RConn1
  Dummy/LConn1 -- Cab Body/RConn1 -- CT/RConn1

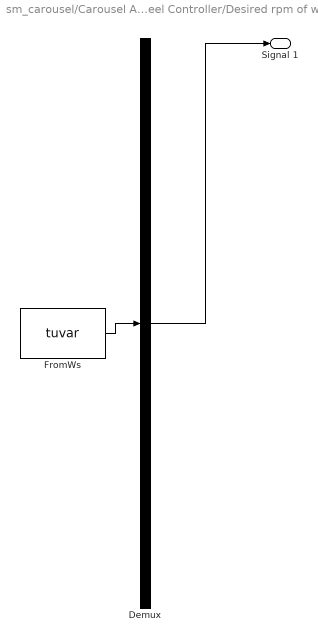
== system sm_carousel/Carousel Assembly/Wheel Controller/Desired rpm of wheel ==
  Demux : Demux  Tag=STV Demux  Outputs=1
      settings: DisplayOption=none
  FromWs : FromWorkspace  Tag=STV FromWs  VariableName=tuvar
      SigBuilderData=|
      | common.afterFinalStr = 'Extrapolate'
      | common.sampleTime = 0
      | dataSet.timeRange = [0 140]
      | dataSet.name = 'Group 1'
      | sbobj.Groups.Name = 'Group 1'
      | sbobj.Groups.Signals.Name = 'Signal 1'
      | sbobj.Groups.Signals.XData = [0 2 22 110 130 140]
      | sbobj.Groups.Signals.YData = [0 0 -15 -15 0 0]
      | sbobj.Groups.TimeRange = [0 140]
  Signal 1 : Outport  Tag=STV Outport
  wires:
  Demux/1 -> Signal 1/1
  FromWs/1 -> Demux/1
